simulink model "ROS_PID"  (R2015b)
settings: Solver=VariableStepAuto  StartTime=0.0  StopTime=60+1  FixedStep=Ts  RelTol=1e-3
values from neighbouring files (symbols this model uses):
  Ts = 0.01    [Plot_interface.m]
undefined symbols (not defined in the file or in its folder): Angular, Discrete, Linear, Time
libraries: robotlib x5, simulink x5, realtime_pacer_lib x4, ctrlSharedLib x1, aerolibtransform2 x1
settings Model: Creator=carlosluis  LastModifiedBy=carlosluis
settings DebuggingCC: MultiTaskRateTransMsg=warning  SingleTaskRateTransMsg=warning

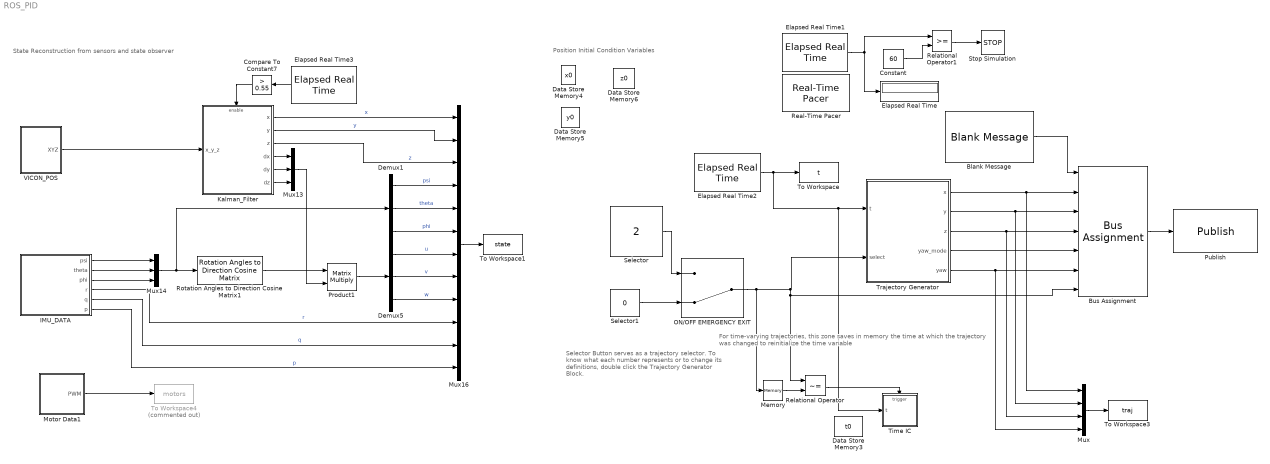
== system ROS_PID ==
  note: State Reconstruction from sensors and state observer
  note: Selector Button serves as a
      | trajectory selector. To know what
      | each number represents or to change its definitions, double click the Trajectory Generator Block.
  note: For time-varying trajectories, this zone saves in memory the
      | time at which the trajectory was changed to reinitialize the time
      | variable
  note: Position Initial Condition Variables
  Blank Message : robotlib/Blank Message  SourceLibraryInfo=This block requires Robotics System Toolbox  messageType=geometry_msgs/Twist  SampleTime=inf
  Bus Assignment : BusAssignment  AssignedSignals=Linear.X,Linear.Y,Linear.Z,Angular.Y,Angular.Z,Angular.X
  Compare To Constant7 : simulink/Logic and Bit Operations/Compare To Constant  relop=>  const=0.55  OutDataTypeStr=boolean
  Constant : Constant  Value=60
  Data Store Memory3 : DataStoreMemory  DataStoreName=t0  ReadBeforeWriteMsg=warning  WriteAfterWriteMsg=warning  WriteAfterReadMsg=warning  OutDataTypeStr=double
  Data Store Memory4 : DataStoreMemory  DataStoreName=x0  ReadBeforeWriteMsg=warning  WriteAfterWriteMsg=warning  WriteAfterReadMsg=warning  OutDataTypeStr=double
  Data Store Memory5 : DataStoreMemory  DataStoreName=y0  ReadBeforeWriteMsg=warning  WriteAfterWriteMsg=warning  WriteAfterReadMsg=warning  OutDataTypeStr=double
  Data Store Memory6 : DataStoreMemory  DataStoreName=z0  ReadBeforeWriteMsg=warning  WriteAfterWriteMsg=warning  WriteAfterReadMsg=warning  OutDataTypeStr=double
  Demux1 : Demux  Outputs=3
  Demux5 : Demux  Outputs=3
  Elapsed Real Time : Display
      settings: Decimation=2
  Elapsed Real Time1 : realtime_pacer_lib/Elapsed Real Time
  Elapsed Real Time2 : realtime_pacer_lib/Elapsed Real Time
  Elapsed Real Time3 : realtime_pacer_lib/Elapsed Real Time
  IMU_DATA : Subsystem
  Kalman_Filter : Subsystem
  Memory : Memory
  Motor Data1 : Subsystem
  Mux : Mux
  Mux13 : Mux  Inputs=3
  Mux14 : Mux  Inputs=3
  Mux16 : Mux  Inputs=12
  ON/OFF EMERGENCY EXIT : ManualSwitch  CurrentSetting=0
  Product1 : Product  Multiplication=Matrix(*)
  Publish : robotlib/Publish  SourceLibraryInfo=This block requires Robotics System Toolbox  topicSource=Specify your own  topic=/goal  messageType=geometry_msgs/Twist  messageQueueLength=1
  Real-Time Pacer : realtime_pacer_lib/Real-Time Pacer  simTimePerRealTime=1
  Relational Operator : RelationalOperator  Operator=~=  OutDataTypeStr=boolean
  Relational Operator1 : RelationalOperator  OutDataTypeStr=boolean
  Rotation Angles to Direction Cosine Matrix1 : aerolibtransform2/Rotation Angles to Direction Cosine Matrix  rotationOrder=ZYX
  Selector : Constant  Value=2
  Selector1 : Constant  Value=0
  Stop Simulation : Stop
  Time IC : Subsystem
  To Workspace : ToWorkspace  VariableName=t  SampleTime=Ts
  To Workspace1 : ToWorkspace  VariableName=state  SampleTime=Ts
  To Workspace3 : ToWorkspace  VariableName=traj  SampleTime=Ts
  To Workspace4 : ToWorkspace  Commented=on  VariableName=motors  SampleTime=Ts
  Trajectory Generator : MATLAB Function  TreatAsAtomicUnit=on
  VICON_POS : Subsystem
  wires:
  Bus Assignment/1 -> Publish/1
  Elapsed Real Time2/1 -> Time IC/1(t), Trajectory Generator/1(t), To Workspace/1
  Blank Message/1 -> Bus Assignment/1
  Memory/1 -> Relational Operator/2
  Relational Operator/1 -> Time IC/Trigger
  Elapsed Real Time1/1 -> Elapsed Real Time/1, Relational Operator1/1
  Trajectory Generator/1(x) -> Bus Assignment/2, Mux/1
  Trajectory Generator/4(yaw_mode) -> Bus Assignment/5
  Trajectory Generator/3(z) -> Bus Assignment/4, Mux/3
  Trajectory Generator/5(yaw) -> Bus Assignment/6, Mux/4
  Trajectory Generator/2(y) -> Bus Assignment/3, Mux/2
  Mux/1 -> To Workspace3/1
  Constant/1 -> Relational Operator1/2
  Relational Operator1/1 -> Stop Simulation/1
  Mux14/1 -> Demux1/1, Rotation Angles to Direction Cosine Matrix1/1
  Rotation Angles to Direction Cosine Matrix1/1 -> Product1/1
  Product1/1 -> Demux5/1
  Elapsed Real Time3/1 -> Compare To Constant7/1
  Compare To Constant7/1 -> Kalman_Filter/Enable
  Kalman_Filter/4(dx) -> Mux13/1
  Kalman_Filter/5(dy) -> Mux13/2
  Kalman_Filter/6(dz) -> Mux13/3
  IMU_DATA/1(psi) -> Mux14/1
  IMU_DATA/2(theta) -> Mux14/2
  IMU_DATA/3(phi) -> Mux14/3
  Mux13/1 -> Product1/2
  Kalman_Filter/1(x) -> Mux16/1  "x"
  Kalman_Filter/2(y) -> Mux16/2  "y"
  Kalman_Filter/3(z) -> Mux16/3  "z"
  IMU_DATA/4(r) -> Mux16/10  "r"
  IMU_DATA/5(q) -> Mux16/11  "q"
  IMU_DATA/6(p) -> Mux16/12  "p"
  Mux16/1 -> To Workspace1/1
  Demux5/1 -> Mux16/7  "u"
  Demux5/2 -> Mux16/8  "v"
  Demux5/3 -> Mux16/9  "w"
  Demux1/1 -> Mux16/4  "psi"
  Demux1/2 -> Mux16/5  "theta"
  Demux1/3 -> Mux16/6  "phi"
  Motor Data1/1(PWM) -> To Workspace4/1
  VICON_POS/1(XYZ) -> Kalman_Filter/1(x_y_z)
  Selector1/1 -> ON/OFF EMERGENCY EXIT/2
  Selector/1 -> ON/OFF EMERGENCY EXIT/1
  ON/OFF EMERGENCY EXIT/1 -> Memory/1, Trajectory Generator/2(select), Bus Assignment/7, Relational Operator/1

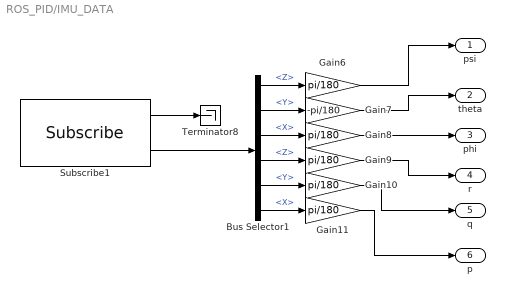
== system ROS_PID/IMU_DATA ==
  Bus Selector1 : BusSelector  OutputSignals=AngularVelocity.Z,AngularVelocity.Y,AngularVelocity.X,LinearAcceleration.Z,LinearAcceleration.Y,LinearAcceleration.X
  Gain{6,8..11} (5 alike) : Gain  Gain=pi/180
  Gain7 : Gain  Gain=-pi/180
  Subscribe1 : robotlib/Subscribe  SourceLibraryInfo=This block requires Robotics System Toolbox  topicSource=Specify your own  topic=/crazyflie/imu  messageType=sensor_msgs/Imu  sampleTime=1/50  messageQueueLength=1
  Terminator8 : Terminator
  psi : Outport
  theta : Outport  Port=2
  phi : Outport  Port=3
  r : Outport  Port=4
  q : Outport  Port=5
  p : Outport  Port=6
  wires:
  Gain11/1 -> p/1
  Gain10/1 -> q/1
  Gain9/1 -> r/1
  Subscribe1/2 -> Bus Selector1/1
  Subscribe1/1 -> Terminator8/1
  Bus Selector1/3 -> Gain8/1  "<X>"
  Bus Selector1/2 -> Gain7/1  "<Y>"
  Bus Selector1/1 -> Gain6/1  "<Z>"
  Bus Selector1/4 -> Gain9/1  "<Z>"
  Bus Selector1/5 -> Gain10/1  "<Y>"
  Bus Selector1/6 -> Gain11/1  "<X>"
  Gain7/1 -> theta/1
  Gain8/1 -> phi/1
  Gain6/1 -> psi/1

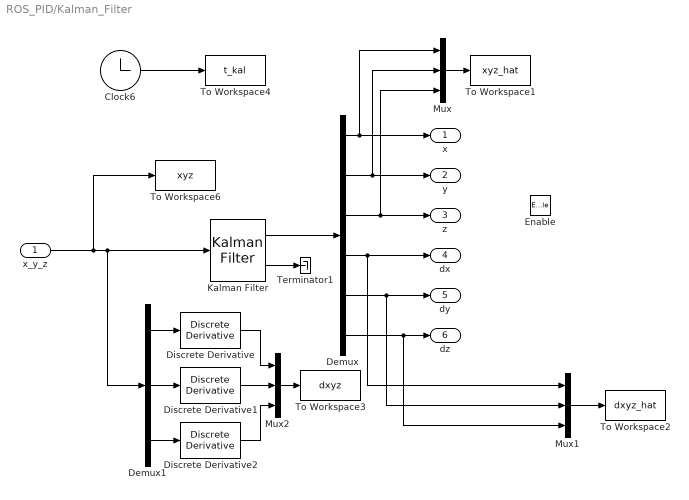
== system ROS_PID/Kalman_Filter ==
  x_y_z : Inport
  Enable : EnablePort
  Clock6 : Clock
  Demux : Demux  Outputs=6
  Demux1 : Demux  Outputs=3
  Discrete Derivative : simulink/Discrete/Discrete Derivative  gainval=1.0  ICPrevScaledInput=0.0  InputProcessing=Inherited  OutMin=[]  OutMax=[]  OutDataType=fixdt(1, 16)  OutScaling=2^-10  DoSatur=off
  Discrete Derivative1 : simulink/Discrete/Discrete Derivative  gainval=1.0  ICPrevScaledInput=0.0  InputProcessing=Inherited  OutMin=[]  OutMax=[]  OutDataType=fixdt(1, 16)  OutScaling=2^-10  DoSatur=off
  Discrete Derivative2 : simulink/Discrete/Discrete Derivative  gainval=1.0  ICPrevScaledInput=0.0  InputProcessing=Inherited  OutMin=[]  OutMax=[]  OutDataType=fixdt(1, 16)  OutScaling=2^-10  DoSatur=off
  Kalman Filter : ctrlSharedLib/Kalman Filter  TimeDomain=Discrete-Time  UseCurrentEstimator=on  ModelSource=Individual A, B, C, D matrices  ModelSourceVariable=ss(0.95,1,1,0,1)  A=[1 0 0 Ts 0 0; 0 1 0 0 Ts 0; 0 0 1 0 0 Ts; 0 0 0 1 0 0; 0 0 0 0 1 0; 0 0 0 0 0 1]  B=1  C=[1 0 0 0 0 0; 0 1 0 0 0 0; 0 0 1 0 0 0]  D=0  NumberOfStates=1  NumberOfInputs=1  NumberOfOutputs=1  InitialEstimateSource=Dialog  X0=0  P0=10  UseK=off  UseGH=on  NumberOfProcessNoiseInputs=1  G=|  TimeInvariantG=on  H=0  TimeInvariantH=on  Q=diag([8e-8 8e-8 8e-8])  TimeInvariantQ=on  R=diag([5e-9 5e-9 5e-9])  TimeInvariantR=on  N=0  TimeInvariantN=on  AddInputPort=off  AddEnablePort=off  OutputEstimatedY=off  OutputP=on  Ts=Ts
      | [Ts/2 0 0
      | ; 0 Ts/2 0; 0 0 Ts/2; 1 0 0; 0 1 0; 0 0 1]
  Mux : Mux  Inputs=3
  Mux1 : Mux  Inputs=3
  Mux2 : Mux  Inputs=3
  Terminator1 : Terminator
  To Workspace1 : ToWorkspace  VariableName=xyz_hat  SampleTime=Ts
  To Workspace2 : ToWorkspace  VariableName=dxyz_hat  SampleTime=Ts
  To Workspace3 : ToWorkspace  VariableName=dxyz  SampleTime=Ts
  To Workspace4 : ToWorkspace  VariableName=t_kal  SampleTime=Ts
  To Workspace6 : ToWorkspace  VariableName=xyz  SampleTime=Ts
  x : Outport
  y : Outport  Port=2
  z : Outport  Port=3
  dx : Outport  Port=4
  dy : Outport  Port=5
  dz : Outport  Port=6
  wires:
  Demux/6 -> Mux1/3, dz/1
  Demux/5 -> Mux1/2, dy/1
  Demux/4 -> Mux1/1, dx/1
  Demux/2 -> Mux/2, y/1
  Demux/3 -> Mux/3, z/1
  Kalman Filter/1 -> Demux/1
  Demux/1 -> Mux/1, x/1
  x_y_z/1 -> To Workspace6/1, Demux1/1, Kalman Filter/1
  Kalman Filter/2 -> Terminator1/1
  Mux/1 -> To Workspace1/1
  Mux1/1 -> To Workspace2/1
  Mux2/1 -> To Workspace3/1
  Clock6/1 -> To Workspace4/1
  Demux1/3 -> Discrete Derivative2/1
  Discrete Derivative2/1 -> Mux2/3
  Demux1/2 -> Discrete Derivative1/1
  Discrete Derivative1/1 -> Mux2/2
  Discrete Derivative/1 -> Mux2/1
  Demux1/1 -> Discrete Derivative/1

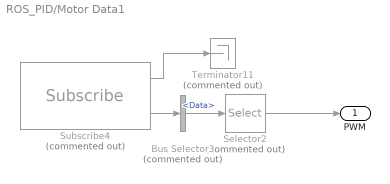
== system ROS_PID/Motor Data1 ==
  Bus Selector3 : BusSelector  Commented=on  OutputSignals=Data
  Selector2 : Selector  Commented=on  InputPortWidth=128  IndexOptions=Index vector (dialog)  Indices=[1 2 3 4]  OutputSizes=1
  Subscribe4 : robotlib/Subscribe  Commented=on  SourceLibraryInfo=This block requires Robotics System Toolbox  topicSource=Specify your own  topic=/crazyflie/motor  messageType=std_msgs/Int32MultiArray  sampleTime=0.1  messageQueueLength=1
  Terminator11 : Terminator  Commented=on
  PWM : Outport
  wires:
  Subscribe4/1 -> Terminator11/1
  Selector2/1 -> PWM/1
  Subscribe4/2 -> Bus Selector3/1
  Bus Selector3/1 -> Selector2/1  "<Data>"

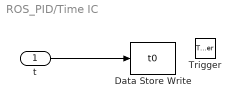
== system ROS_PID/Time IC ==
  t : Inport
  Trigger : TriggerPort  PortDimensions=1
  Data Store Write : DataStoreWrite  DataStoreName=t0
  wires:
  t/1 -> Data Store Write/1

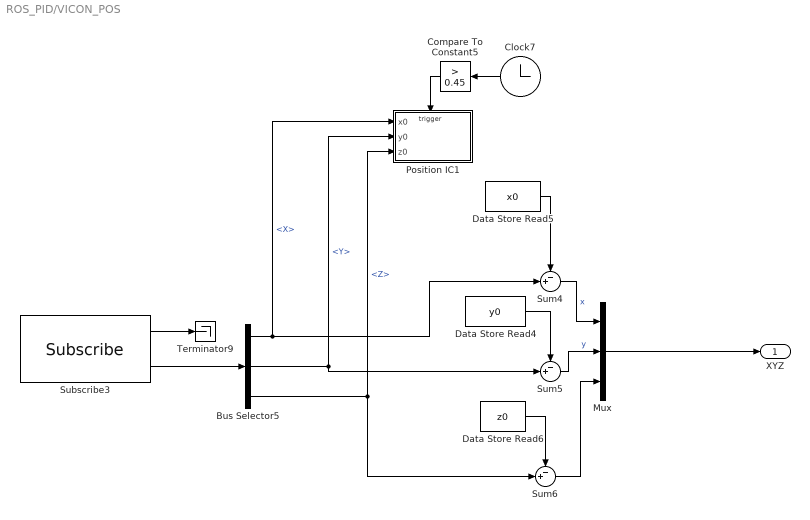
== system ROS_PID/VICON_POS ==
  Bus Selector5 : BusSelector  OutputSignals=X,Y,Z
  Clock7 : Clock
  Compare To Constant5 : simulink/Logic and Bit Operations/Compare To Constant  relop=>  const=0.45  OutDataTypeStr=boolean
  Data Store Read4 : DataStoreRead  DataStoreName=y0  SampleTime=Ts
  Data Store Read5 : DataStoreRead  DataStoreName=x0  SampleTime=Ts
  Data Store Read6 : DataStoreRead  DataStoreName=z0  SampleTime=Ts
  Mux : Mux  Inputs=3
  Position IC1 : Subsystem
  Subscribe3 : robotlib/Subscribe  SourceLibraryInfo=This block requires Robotics System Toolbox  topicSource=Specify your own  topic=/vicon/pos  messageType=geometry_msgs/Vector3  sampleTime=Ts  messageQueueLength=1
  Sum4 : Sum  Inputs=-+|
  Sum5 : Sum  Inputs=-+|
  Sum6 : Sum  Inputs=-+|
  Terminator9 : Terminator
  XYZ : Outport
  wires:
  Bus Selector5/2 -> Sum5/2, Position IC1/2(y0)  "<Y>"
  Bus Selector5/1 -> Sum4/2, Position IC1/1(x0)  "<X>"
  Bus Selector5/3 -> Sum6/2, Position IC1/3(z0)  "<Z>"
  Subscribe3/2 -> Bus Selector5/1
  Subscribe3/1 -> Terminator9/1
  Compare To Constant5/1 -> Position IC1/Trigger
  Clock7/1 -> Compare To Constant5/1
  Data Store Read5/1 -> Sum4/1
  Data Store Read4/1 -> Sum5/1
  Data Store Read6/1 -> Sum6/1
  Sum4/1 -> Mux/1  "x"
  Sum5/1 -> Mux/2  "y"
  Mux/1 -> XYZ/1
  Sum6/1 -> Mux/3

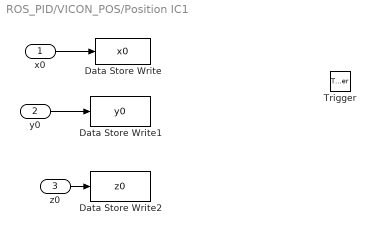
== system ROS_PID/VICON_POS/Position IC1 ==
  x0 : Inport
  y0 : Inport  Port=2
  z0 : Inport  Port=3
  Trigger : TriggerPort  PortDimensions=1
  Data Store Write : DataStoreWrite  DataStoreName=x0
  Data Store Write1 : DataStoreWrite  DataStoreName=y0
  Data Store Write2 : DataStoreWrite  DataStoreName=z0
  wires:
  x0/1 -> Data Store Write/1
  y0/1 -> Data Store Write1/1
  z0/1 -> Data Store Write2/1

== matlab function ROS_PID/Trajectory Generator ==
  data: x output; t input; y output; z output; yaw_mode output; yaw output; select input; t0 data_store_memory
function [x,y,z,yaw_mode,yaw] = message(t,select)
x = 0;
y= 0;
z = 0;
yaw_mode = 0; % 0 for Position mode, 1 for Rate mode
yaw = 0; %If position mode, then this is the setpoint in deg
         %If rate mode, then the setpoint is in deg/s
global t0; 
switch(select) 
    case 1 %PROTECTED case, left unchanged for landing
        x= 0;
        y= 0;
        z= -0.1*(t-t0); %specify rate in cm/s for descending
        yaw_mode = 0;
        yaw=0;   
               
    case 2 % Hover 1 meter altitude @ initial position
        
        if(t<12)
        x = 0; %The initial position is always added ROS side
        y = 0; %Same here, x_0 and y_0 are automatically added in ROS  
        z = 1;
        yaw_mode = 0;
        yaw = 0;
        end
        
        if(t>12 & t<25)
        x = 0;
        y = 0;
        z = 2;
        yaw_mode = 0;
        yaw = 0;
        end
        
        if(t>25)
        x = 0;
        y = 0; 
        z = 1;
        yaw_mode = 0;
        yaw = 0;
        end
        
    case 3 %Step in the X direction
        x = 0;
        y = 0;
        z = 1;
        yaw_mode = 0;
        yaw = 0;
        
    case 4 %Circular trajectory @ 1m altitude and constant yaw velocity
       if(t<10)
        x = 0; 
        y = 0;
        z = 1;
        yaw_mode = 0;
        yaw = 0;
       end
        
       if(t>10 & t<50)
        w = 0.1;
        x = sin(2*pi*w*(t-10));
        y = sin(2*pi*w*(t-10) + pi/2);
        z = 1;
        yaw_mode = 1; %Rate mode
        yaw = 90;
       end
       
       if(t>50)
        x = 0; 
        y = 0;  
        z = 1;
        yaw_mode = 0;
        yaw = 0;
       end
        
    case 5 %Helical trajectory and constant yaw velocity 
        if(t<40)
        w = 0.1;
        x = 0.8*sin(2*pi*w*(t-t0));
        y = 0.8*sin(2*pi*w*(t-t0) + pi/2);
        z=  0.4 + 0.04*(t-t0);
        yaw_mode = 1; %Rate mode
        yaw = 60;           
        end
        
        if(t>40 & t<50)
        x = 0; 
        y = 0;  
        z = 1;
        yaw_mode = 0;
        yaw = 0;
        end
        
        if(t>50)
        x= 0;
        y= 0;
        z= -0.1*(t-50); %specify rate in cm/s for descending
        yaw_mode = 0;
        yaw=0;   
        end
       
        
    otherwise
          x= 0;
          y= 0;
          z= 0;
          yaw_mode = 0;
          yaw=0;
     
end
end
